simulink model "RR_Thrust_Forces"  (R2023b)
settings: Solver=VariableStepAuto  StartTime=0.0  StopTime=10.0  RelTol=1e-3
values from neighbouring files (symbols this model uses):
  RR_Motors_Thrust = [4.04656097579 98.9159349639]    [RR.mat]
  RR_Motors_Thrust_Alt_Lut = [0 10000 20000 30000]    [RR.mat]
  RR_Motors_Thrust_Pct_Lut = [1 0.705882352941 0.470588235294 0.352941176471]    [RR.mat]
settings Model: Creator=jrighetti  LastModifiedBy=jrighetti

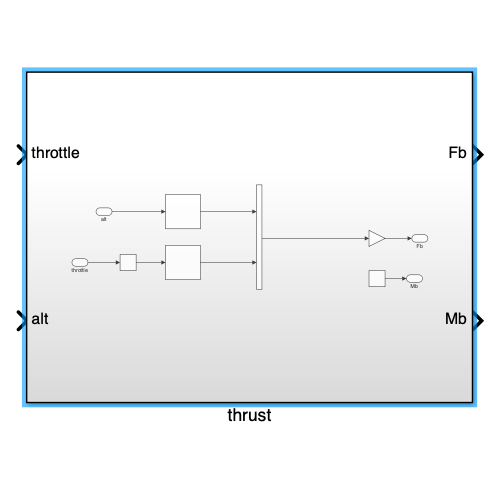
[thumbnail: Simulink's stored preview of the top-level diagram]
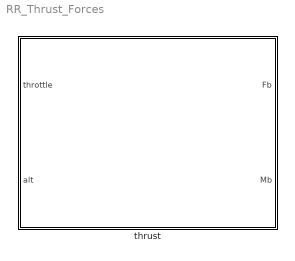
== system RR_Thrust_Forces ==
  thrust : Subsystem

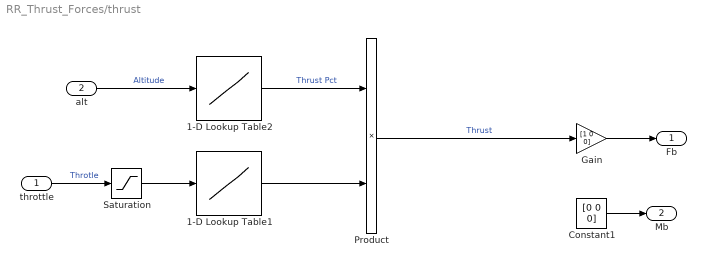
== system RR_Thrust_Forces/thrust ==
  throttle : Inport
  alt : Inport  Port=2
  1-D Lookup Table1 : Lookup_n-D  NumberOfTableDimensions=1  BreakpointsForDimension1=[0,1]  Table=RR_Motors_Thrust  InternalRulePriority=Speed  RndMeth=Simplest
  1-D Lookup Table2 : Lookup_n-D  NumberOfTableDimensions=1  BreakpointsForDimension1=RR_Motors_Thrust_Alt_Lut  Table=RR_Motors_Thrust_Pct_Lut  InternalRulePriority=Speed  RndMeth=Simplest
  Constant1 : Constant  Value=[0 0 0]
  Gain : Gain  Gain=[1 0 0]
  Product : Product
  Saturation : Saturate  UpperLimit=1.0  LowerLimit=0.0
  Fb : Outport
  Mb : Outport  Port=2
  wires:
  throttle/1 -> Saturation/1  "Throtle"
  alt/1 -> 1-D Lookup Table2/1  "Altitude"
  1-D Lookup Table2/1 -> Product/1  "Thrust Pct"
  1-D Lookup Table1/1 -> Product/2
  Saturation/1 -> 1-D Lookup Table1/1
  Product/1 -> Gain/1  "Thrust"
  Gain/1 -> Fb/1
  Constant1/1 -> Mb/1
